simulink model "FeedbackData"  (Simulink 7.6)
settings: Solver=FixedStepDiscrete  StartTime=0.0  StopTime=runTime  FixedStep=dt  RelTol=1e-3
values from neighbouring files (symbols this model uses):
  dataSize = hmDataSize + rigidBodies*rigidBodyDataSize + markers*markerDataSize    (= 111)    [initCode.m]
  dt = 1/52    (= 0.0192307692308)    [initCode.m]    (also in logdata.m)
  hypx = modeldata.muscle(10).Fx.hyp.cov    [initCode.m]
  hypy = modeldata.muscle(10).Fy.hyp.cov    [initCode.m]
  hypz = modeldata.muscle(10).Fz.hyp.cov    [initCode.m]
  Ki = 0    [initCode.m]
  Kp = 0    [initCode.m]
  KXX_x = (KXX+sigma2*eye(size(KXX,1)))    [initCode.m]
  KXX_y = (KXX+sigma2*eye(size(KXX,1)))    [initCode.m]
  KXX_z = (KXX+sigma2*eye(size(KXX,1)))    [initCode.m]
  M = data(idx).M    [initCode.m]
  maxF = [max(trainingOutputs_x),max(trainingOutputs_y),max(trainingOutputs_z)]    [initCode.m]
  minF = [min(trainingOutputs_x),min(trainingOutputs_y),min(trainingOutputs_z)]    [initCode.m]
  pwmat = [0 0 0 0 0 0 0 0 0;250 23 10 20 49 62 107 22 25]    [initCode.m]
  rcparams = zeros(9,4)    [initCode.m]
  runTime = 5    [initCode.m]
  stimStartTime = 0.1    [initCode.m]
  trainingInputs = modeldata.muscle(10).Fx.trainingInputs    [initCode.m]
  trainingOutputs_x = modeldata.muscle(10).Fx.trainingOutputs    [initCode.m]
  trainingOutputs_y = modeldata.muscle(10).Fy.trainingOutputs    [initCode.m]
  trainingOutputs_z = modeldata.muscle(10).Fz.trainingOutputs    [initCode.m]
  trajectory = [data(idx).traj(:,1:3) data(idx).t(:,1:3) data(idx).forceRange]    [initCode.m]
undefined symbols (not defined in the file or in its folder): DiscIntNeverNeededParam, Implant, IST
libraries: xpclib x8, devices x5, FreqBlockset x2, simulink x1
settings Model: Creator=Engineer  LastModifiedBy=KirschLab  BufferReuse=off
settings DataIOCC: LimitDataPoints=off  SaveFormat=StructureWithTime  SignalLogging=off
settings OptimizationCC: BlockReduction=off  OptimizeBlockIOStorage=off  BufferReuse=off  ExpressionFolding=off  LocalBlockOutputs=off  InitFltsAndDblsToZero=on  SimCompilerOptimization=On
settings DebuggingCC: StrictBusMsg=Warning
settings HardwareCC: ProdIntDivRoundTo=Zero  ProdEndianess=LittleEndian  ProdHWDeviceType=Generic->32-bit x86 compatible  TargetHWDeviceType=32-bit Generic
settings RTWCC: SystemTargetFile=xpctarget.tlc  TemplateMakefile=xpc_default_tmf  Description=xPC Target  ProcessScript=xpctarget_make_rtw_hook  RTWCompilerOptimization=On
settings xpcTargetCC: TargetFcnLib=ansi_tfl_table_tmw.mat  TargetFunctionLibrary=XPC_BLAS  ERTCodeCoverageTool=None  ParMdlRefBuildCompliant=on  CombineSignalStateStructs=off  PortableWordSizes=off  xPCLoadParamSetFile=off  xPCConcurrentTasks=off  xPCEnableSFAnimation=off

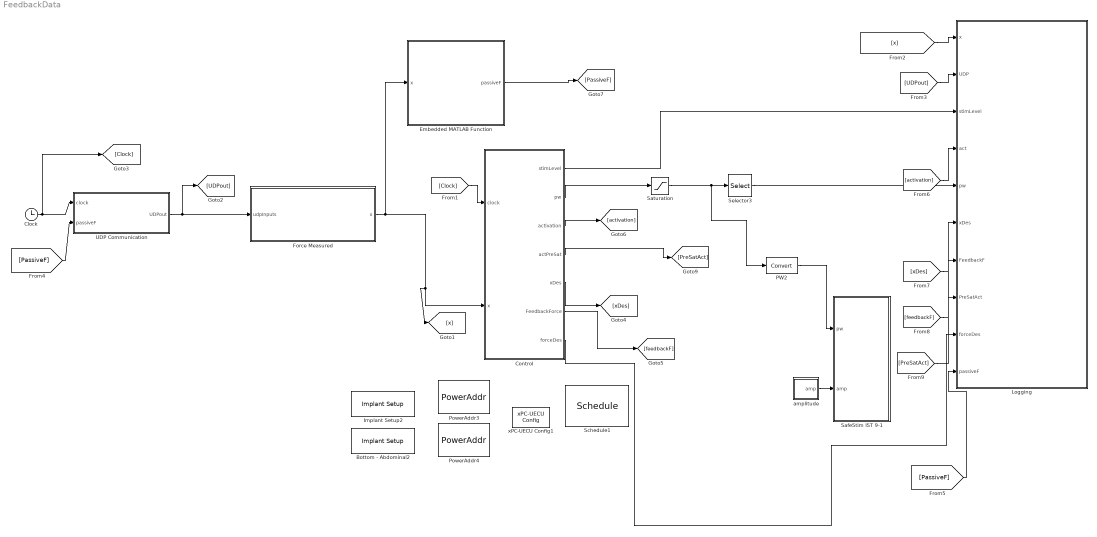
== system FeedbackData ==
  Bottom - Abdominal2 : devices/Implant Setup  implant=IST-12  addr=Implant(2).Addr  port=Implant(2).Port  id=0  hs=off  dup=off
  Clock : Clock
      settings: Decimation=10
  Control : Subsystem  TreatAsAtomicUnit=on
  Embedded MATLAB Function : Stateflow chart  TreatAsAtomicUnit=on
  Force Measured : Subsystem
  Implant Setup2 : devices/Implant Setup  implant=IST-12  addr=Implant(1).Addr  port=Implant(1).Port  id=0  hs=off  dup=off
  Logging : Subsystem
  PW2 : DataTypeConversion
  PowerAddr3 : FreqBlockset/Schedule_Setup/PowerAddr  SystemSampleTime=-1  rf_power=Implant(1).Power  addr=Implant(1).Addr  sched_T=uecuFreq  port=Implant(1).Port
  PowerAddr4 : FreqBlockset/Schedule_Setup/PowerAddr  SystemSampleTime=-1  rf_power=Implant(2).Power  addr=Implant(2).Addr  sched_T=uecuFreq  port=Implant(2).Port
  SafeStim IST 9-1 : Subsystem  mask{addr=Implant(2).Addr, port=Implant(2).Port, chvector=[0 1 2 3 4 5 6 7 8 9 10 11], alimits=[4 4 2 3 2 3 2 2 3 5 5 8], dvector=[10 11 12 13 14 15 16 17 18 19 20 21], schedulename=schedule1, spriority=100, Tsamp=-1}
      mask prompts: addr "Address"; chvector "Channel Vector"; alimits "Amplitude Level Limits"; dvector "Delay vector (ms)"; schedulename "Schedule name"; spriority "Scheduler priority"; Tsamp "Sample time (s) (Update rate.  Pulse period is set by Schedule block.)"
      mask CallbackString: |||||set_param([gcb '/Stim'],'sched',get_param(gcb,'schedulename'))||
      mask Display:
      | fprintf('Safe Stimulation\nSet Amp Limits')
      | port_label('input',1,'pw(us)')
      | port_label('input',2,'amp(level)')
  Saturation : Saturate  UpperLimit=250  LowerLimit=0
  Schedule1 : devices/Schedule  sched=schedule1  stype=Synchronous  period=80  t=1/13
  Selector3 : Selector  InputPortWidth=12  IndexOptions=Index vector (dialog)  Indices=[1 2 3 4 7 9 10 11 12]  OutputSizes=1
  UDP Communication : Subsystem
  amplitude : Subsystem
  xPC-UECU Config1 : devices/xPC Functions/xPC-UECU Config  port=COM1  baud=115200  flowctrl=on  addr=128
  wires:
  [UDPout] -> Logging/2(UDP)
  Control/1(stimLevel) -> Logging/3(stimLevel)
  Control/2(pw) -> Saturation/1
  Saturation/1 -> PW2/1, Selector3/1
  [Clock] -> Control/1(clock)
  Control/3(activation) -> [activation]
  PW2/1 -> SafeStim IST 9-1/1(pw)
  amplitude/1(amp) -> SafeStim IST 9-1/2(amp)
  [x] -> Logging/1(x)
  [activation] -> Logging/4(act)
  Selector3/1 -> Logging/5(pw)
  UDP Communication/1(UDPout) -> [UDPout], Force Measured/1(udpInputs)
  Clock/1 -> UDP Communication/1(clock), [Clock]
  [feedbackF] -> Logging/7(FeedbackF)
  [xDes] -> Logging/6(xDes)
  Control/4(actPreSat) -> [PreSatAct]
  [PreSatAct] -> Logging/8(PreSatAct)
  Control/5(xDes) -> [xDes]
  Force Measured/1(x) -> Control/2(x), [x], Embedded MATLAB Function/1(x)
  Control/6(FeedbackForce) -> [feedbackF]
  Control/7(forceDes) -> Logging/9(forceDes)
  Embedded MATLAB Function/1(passiveF) -> [PassiveF]
  [PassiveF] -> UDP Communication/2(passiveF)
  [PassiveF] -> Logging/10(passiveF)

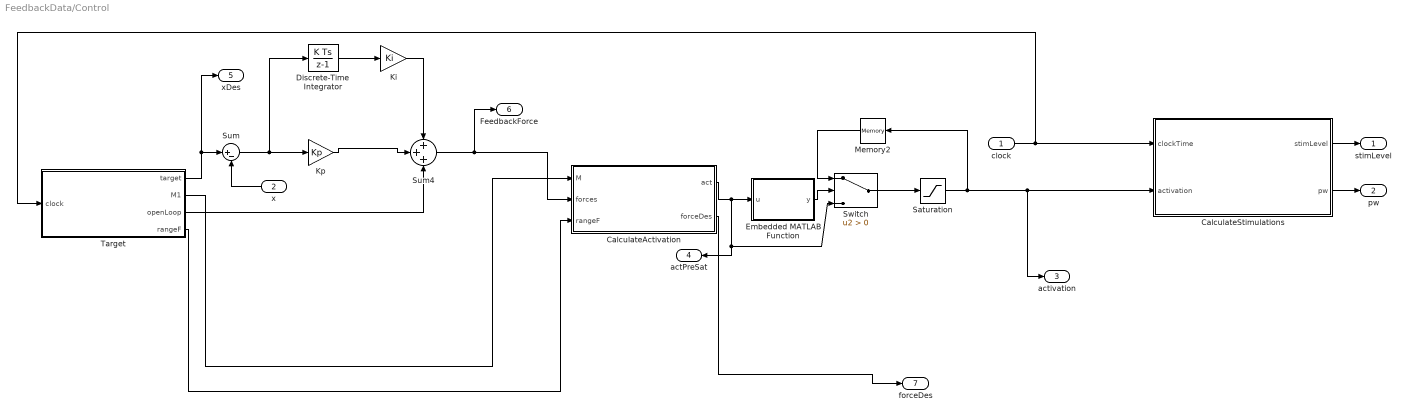
== system FeedbackData/Control ==
  clock : Inport
  x : Inport  Port=2
  CalculateActivation : Stateflow chart  TreatAsAtomicUnit=on
  CalculateStimulations : Stateflow chart  TreatAsAtomicUnit=on
  Discrete-Time Integrator : DiscreteIntegrator  InitialCondition=[0;0;0]  SampleTime=dt  LimitOutput=on  UpperSaturationLimit=[50;50;50]  LowerSaturationLimit=[-50;-50;-50]  ICPrevOutput=DiscIntNeverNeededParam  ICPrevScaledInput=DiscIntNeverNeededParam
  Embedded MATLAB Function : Stateflow chart  TreatAsAtomicUnit=on
  Ki : Gain  Gain=Ki
  Kp : Gain  Gain=Kp
  Memory2 : Memory  X0=[0;0;0;0;0;0;0;0;0]
  Saturation : Saturate  UpperLimit=1  LowerLimit=0
  Sum : Sum  Inputs=|+-
  Sum4 : Sum  Inputs=+++
  Switch : Switch  Criteria=u2 > Threshold
  Target : Stateflow chart  TreatAsAtomicUnit=on
  stimLevel : Outport
  pw : Outport  Port=2
  activation : Outport  Port=3
  actPreSat : Outport  Port=4
  xDes : Outport  Port=5
  FeedbackForce : Outport  Port=6
  forceDes : Outport  Port=7
  wires:
  CalculateStimulations/2(pw) -> pw/1
  CalculateStimulations/1(stimLevel) -> stimLevel/1
  clock/1 -> CalculateStimulations/1(clockTime), Target/1(clock)
  CalculateActivation/1(act) -> Switch/3, actPreSat/1, Embedded MATLAB Function/1(u)
  Saturation/1 -> activation/1, CalculateStimulations/2(activation), Memory2/1
  Memory2/1 -> Switch/1
  Embedded MATLAB Function/1(y) -> Switch/2
  Switch/1 -> Saturation/1
  Target/1(target) -> Sum/1, xDes/1
  x/1 -> Sum/2
  Sum/1 -> Kp/1, Discrete-Time Integrator/1
  Discrete-Time Integrator/1 -> Ki/1
  Ki/1 -> Sum4/1
  Kp/1 -> Sum4/2
  Sum4/1 -> CalculateActivation/2(forces), FeedbackForce/1
  Target/2(M1) -> CalculateActivation/1(M)
  Target/3(openLoop) -> Sum4/3
  Target/4(rangeF) -> CalculateActivation/3(rangeF)
  CalculateActivation/2(forceDes) -> forceDes/1

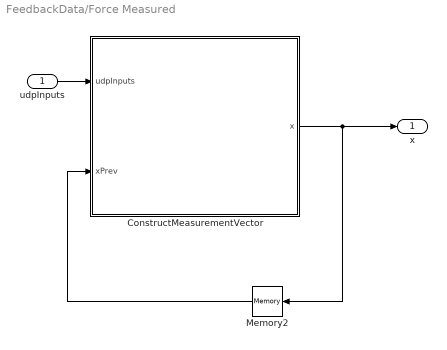
== system FeedbackData/Force Measured ==
  udpInputs : Inport
  ConstructMeasurementVector : Stateflow chart  TreatAsAtomicUnit=on
  Memory2 : Memory  X0=[0;0;0]
  x : Outport
  wires:
  udpInputs/1 -> ConstructMeasurementVector/1(udpInputs)
  ConstructMeasurementVector/1(x) -> x/1, Memory2/1
  Memory2/1 -> ConstructMeasurementVector/2(xPrev)

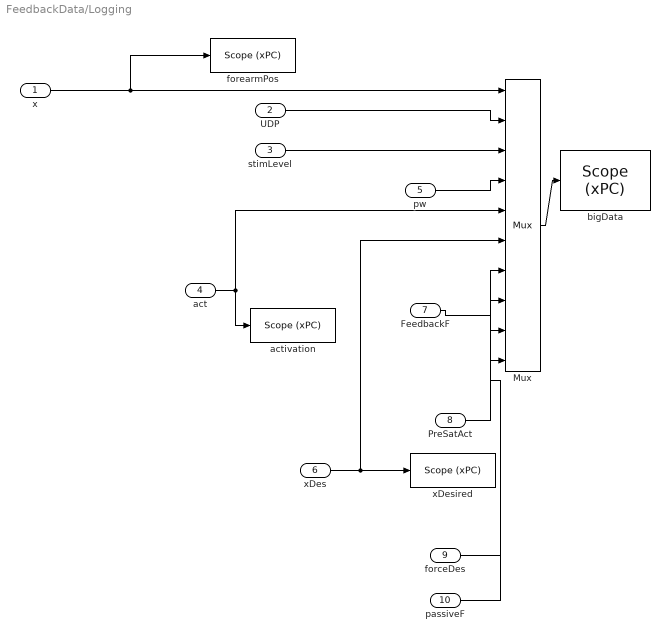
== system FeedbackData/Logging ==
  x : Inport
  UDP : Inport  Port=2
  stimLevel : Inport  Port=3
  act : Inport  Port=4
  pw : Inport  Port=5
  xDes : Inport  Port=6
  FeedbackF : Inport  Port=7
  PreSatAct : Inport  Port=8
  forceDes : Inport  Port=9
  passiveF : Inport  Port=10
  Mux : Mux  Inputs=10
  activation : xpclib/Misc./Scope (xPC)   SystemSampleTime=-1  scopeno=5  scopetype=Target  autostart=on  viewmode=Numerical  formatstr='%15.6f'  grid=on  ylimits=[-1,1]  nosamples=3  noprepostsamples=-50  interleave=1  triggermode=FreeRun  triggersignal=2  triggerlevel=0.5  triggerslope=Either  triggerscope=1  triggersample=0  filename=data.dat  mode=Lazy  writesize=512  autorestart=off  dynamicfilemode=off  maxwritefilesize=512*1024^2
  bigData : xpclib/Misc./Scope (xPC)   SystemSampleTime=-1  scopeno=1  scopetype=File  autostart=on  viewmode=Numerical  formatstr='%15.6f'  grid=on  ylimits=[-1,1]  nosamples=10000  noprepostsamples=-50  interleave=dec  triggermode=FreeRun  triggersignal=2  triggerlevel=0.5  triggerslope=Either  triggerscope=1  triggersample=0  filename=data3.dat  mode=Lazy  writesize=512  autorestart=off  dynamicfilemode=off  maxwritefilesize=512*1024^2
  forearmPos : xpclib/Misc./Scope (xPC)   SystemSampleTime=-1  scopeno=3  scopetype=Target  autostart=on  viewmode=Numerical  formatstr='%15.6f'  grid=on  ylimits=[-1,1]  nosamples=3  noprepostsamples=-50  interleave=1  triggermode=FreeRun  triggersignal=2  triggerlevel=0.5  triggerslope=Either  triggerscope=1  triggersample=0  filename=data.dat  mode=Lazy  writesize=512  autorestart=off  dynamicfilemode=off  maxwritefilesize=512*1024^2
  xDesired : xpclib/Misc./Scope (xPC)   SystemSampleTime=-1  scopeno=4  scopetype=Target  autostart=on  viewmode=Numerical  formatstr='%15.6f'  grid=on  ylimits=[-1,1]  nosamples=3  noprepostsamples=-50  interleave=1  triggermode=FreeRun  triggersignal=2  triggerlevel=0.5  triggerslope=Either  triggerscope=1  triggersample=0  filename=data.dat  mode=Lazy  writesize=512  autorestart=off  dynamicfilemode=off  maxwritefilesize=512*1024^2
  wires:
  act/1 -> activation/1, Mux/5
  pw/1 -> Mux/4
  Mux/1 -> bigData/1
  x/1 -> Mux/1, forearmPos/1
  UDP/1 -> Mux/2
  stimLevel/1 -> Mux/3
  xDes/1 -> xDesired/1, Mux/6
  FeedbackF/1 -> Mux/7
  PreSatAct/1 -> Mux/8
  forceDes/1 -> Mux/9
  passiveF/1 -> Mux/10

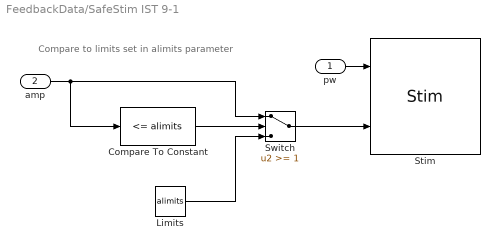
== system FeedbackData/SafeStim IST 9-1 ==
  note: Compare to limits set in alimits parameter
  pw : Inport
  amp : Inport  Port=2
  Compare To Constant : simulink/Logic and Bit Operations/Compare To Constant  SystemSampleTime=-1  relop=<=  const=alimits  LogicOutDataTypeMode=uint8  ZeroCross=off
  Limits : Constant  Value=alimits  OutDataTypeStr=uint8  SampleTime=Tsamp
  Stim : devices/Stim  addr=addr  port=port  chan=chvector  dselect=Parameter  delays=dvector  autosched=Manual  sched=schedule1  pri=spriority  period=Tsamp
  Switch : Switch  Threshold=1  SampleTime=Tsamp
  wires:
  pw/1 -> Stim/1
  amp/1 -> Compare To Constant/1, Switch/1
  Compare To Constant/1 -> Switch/2
  Limits/1 -> Switch/3
  Switch/1 -> Stim/2

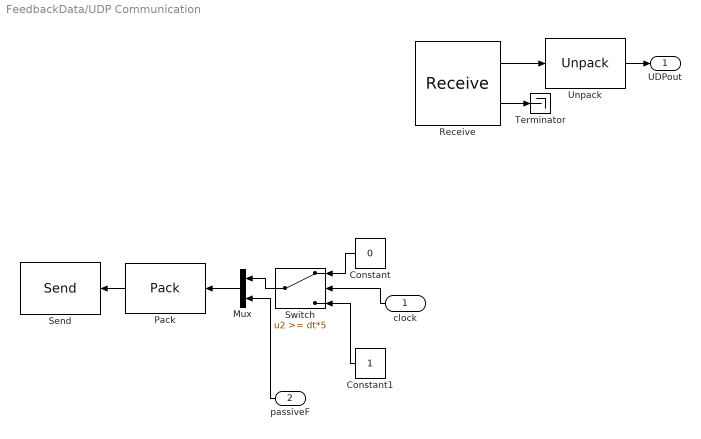
== system FeedbackData/UDP Communication ==
  clock : Inport
  passiveF : Inport  Port=2
  Constant : Constant  Value=0
  Constant1 : Constant
  Mux : Mux  Inputs=2
  Pack : xpclib/UDP/Pack  datatypes={'double'}  byteAlign=1
  Receive : xpclib/UDP/Receive  ipAddress=192.168.0.8  ipPort=25000  width=8*dataSize  vblLen=off  sampletime=dt
  Send : xpclib/UDP/Send  ipAddress=192.168.0.8  ipPort=20000  localPort=-1  vblLen=off  sampletime=dt
  Switch : Switch  Threshold=dt*5
  Terminator : Terminator
  Unpack : xpclib/UDP/Unpack  dimensions={[dataSize]}  datatypes={'double'}  byteAlign=1
  UDPout : Outport
  wires:
  Receive/2 -> Terminator/1
  Receive/1 -> Unpack/1
  Pack/1 -> Send/1
  clock/1 -> Switch/2
  Constant/1 -> Switch/1
  Constant1/1 -> Switch/3
  Unpack/1 -> UDPout/1
  Mux/1 -> Pack/1
  Switch/1 -> Mux/1
  passiveF/1 -> Mux/2

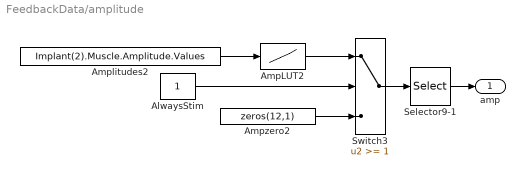
== system FeedbackData/amplitude ==
  AlwaysStim : Constant
  AmpLUT2 : Lookup  InputValues=Implant(2).Muscle.Amplitude.AmpIndices(:,1)  Table=Implant(2).Muscle.Amplitude.AmpIndices(:,2)  LookUpMeth=Interpolation-Use End Values  OutDataTypeStr=uint8  SaturateOnIntegerOverflow=on
  Amplitudes2 : Constant  Value=Implant(2).Muscle.Amplitude.Values  OutDataTypeStr=double
  Ampzero2 : Constant  Value=zeros(12,1)  OutDataTypeStr=uint8
  Selector9-1 : Selector  InputPortWidth=12  IndexOptions=Index vector (dialog)  Indices=[1 2 3 4 5 6 7 8 9 10 11 12]  OutputSizes=1
  Switch3 : Switch  Threshold=1
  amp : Outport
  wires:
  Amplitudes2/1 -> AmpLUT2/1
  Ampzero2/1 -> Switch3/3
  Switch3/1 -> Selector9-1/1
  AmpLUT2/1 -> Switch3/1
  AlwaysStim/1 -> Switch3/2
  Selector9-1/1 -> amp/1

== matlab function Control/Embedded MATLAB Function ==
  data: u input double; y output double
function y = fcn(u)
%#eml

y = sum(isnan(u));

== matlab function Control/Target ==
  data: trajectory parameter double; M parameter double; target output double; clock input double; runTime parameter double; M1 output double; openLoop output double; rangeF output double
function [target,M1,openLoop,rangeF]   = calcTarget(trajectory,M,clock,runTime)
%#eml

dt=1/52;
steps=runTime/dt;
idx=floor(clock/runTime*steps)+1;
if idx>length(trajectory)
    idx=length(trajectory);
end


target=trajectory(idx,1:3)';
openLoop=trajectory(idx,4:6)';
M1=M(:,:,idx);
rangeF=trajectory(idx,7:12)';

== matlab function Force Measured/ConstructMeasurementVector ==
  data: udpInputs input double; x output double; xPrev input double
function x    = cmv(udpInputs,xPrev)
%#eml


forearmFlagIndex = 39;

forearmFlag = udpInputs(forearmFlagIndex); 
if forearmFlag % if the forearm rigid body is visiable record the sensor readings
	x = udpInputs(36:38); 
else 
    x=xPrev;
end

== matlab function Control/CalculateActivation ==
  data: M input double; act output double; forces input double; actDesired parameter double; rangeF input double; forceDes output double
function [act,forceDes]  = computeActivations(M,forces,actDesired,rangeF)
%#eml

% % solve Malpha=forces for alpha


% Use desired activation if previous activations were too high or low
% This should help stop the solution from running away

x=actDesired;
normal = [0 0 1; 0 0 -1; -1 0 0; 1 0 0; 0 1 0; 0 -1 0];

forceDes=forces;
Fdes=forceDes;
unitvector=Fdes';
% Make norm of forces small if needed
% Method by Zinnia Hall
xyz_max=rangeF([2 4 6]);
xyz_min=rangeF([1 3 5]);
if Fdes(1)> xyz_max(1) || Fdes(2)> xyz_max(2) || Fdes(3)> xyz_max(3) || Fdes(1)< xyz_min(1) || Fdes(2)< xyz_min(2) || Fdes(3)< xyz_min(3)
    xyz_plane1 = [xyz_min(1) xyz_min(2) xyz_max(3)];
    xyz_plane2 = [xyz_min(1) xyz_min(2) xyz_min(3)];
    xyz_plane3 = [xyz_min(1) xyz_max(2) xyz_max(3)];
    xyz_plane4 = [xyz_max(1) xyz_min(2) xyz_min(3)];
    xyz_plane5 = [xyz_max(1) xyz_max(2) xyz_max(3)];
    xyz_plane6 = [xyz_max(1) xyz_min(2) xyz_max(3)];
    d1 = (dot((xyz_plane1 - zeros(1,3)),normal(1,:)))/(dot(unitvector,normal(1,:)));
    d2 = (dot((xyz_plane2 - zeros(1,3)),normal(2,:)))/(dot(unitvector,normal(2,:)));
    d3 = (dot((xyz_plane3 - zeros(1,3)),normal(3,:)))/(dot(unitvector,normal(3,:)));
    d4 = (dot((xyz_plane4 - zeros(1,3)),normal(4,:)))/(dot(unitvector,normal(4,:)));
    d5 = (dot((xyz_plane5 - zeros(1,3)),normal(5,:)))/(dot(unitvector,normal(5,:)));
    d6 = (dot((xyz_plane6 - zeros(1,3)),normal(6,:)))/(dot(unitvector,normal(6,:)));
    % ratio of perpendicular distance between point on plane vector and infeasible vector
    distance = [d1 d2 d3 d4 d5 d6];
    distance = distance(distance>=0); %creates vector with positive values
    distance = min(distance);
    point = (distance*unitvector)+zeros(1,3);
    Fdes_new = point; % Point of intersection with plane
    forceDes=Fdes_new';
end

forces=forceDes;
Bk=eye(9);
func=@penaltyFunc;
[f,g]=func(x,M,forces);

it=0;
while norm(g)>1e-3 && it<120
    p=-Bk*g;
    alpha2=armijo(func,x,f,g,p,M,forces);
    xold=x;
    x=x+alpha2*p;
    sk=x-xold;
    gold=g;
    [f,g]=func(x,M,forces);
    yk=g-gold;
    rho=1/(yk'*sk);
    Bk=(eye(9)-rho*sk*yk')*Bk*(eye(9)-rho*yk*sk')+rho*sk*sk';
    it=it+1;
end

if max(x)>1
    x=x/max(x);
end


act=x;
end

function alpha1 = armijo(func,xk,fk,gradk,pk,M,forces)
% Originally from Dr. Schearer. Modified by Derek Wolf
alpha1   = 1;
c       = 0;
rho     = 0.5;

n=0;
while fk + c*alpha1*gradk'*pk < func(xk+alpha1*pk,M,forces) % sufficient descent condition is not met
    alpha1 = rho*alpha1;
    n=n+1;
end
end

function [f,g]=penaltyFunc(x,M,forces)
c3 = 1000;
c2 = 10000;
c1 = 100;

K=0;
for i=1:length(x)
    if x(i)<0
        K=K+x(i)^2;
    end
    if x(i)>1
        K = K + (x(i)-1)^2;
    end
end

dirConst = [forces(2)*M(3,:)-forces(3)*M(2,:);forces(3)*M(1,:)-forces(1)*M(3,:);forces(1)*M(2,:)-forces(2)*M(1,:)];
f=norm(x)^2+c1*norm(M*x-forces)^2+c2*K + c3*norm(dirConst*x)^2;

if nargout>1
    % Define gradient
    K=zeros(9,1);
    for i=1:length(x)
        if x(i)<0
            K(i)=2*x(i);
        end
        if x(i) > 1
            K(i) = 2*(x(i)-1);
        end
    end
    
    g = 2*x + 2*c1*M'*(M*x-forces) + c2*K + 2*c3*dirConst'*dirConst*x;
end


end

% function [f,g]=penaltyFunc(x,M,forces)
%
% c2=5000;
% c=1;
%
%
% K=0;
% for i=1:length(x)
%     if x(i)<0
%         K=K+x(i)^2;
%     end
% end
%
% f=c*norm(x)^2+norm(M*x-forces)^2+c2*K;
%
% if nargout>1
%     % Define gradient
%     K=zeros(9,1);
%     for i=1:length(x)
%         if x(i)<0
%             K(i)=2*x(i);
%         end
%     end
%
%     g=c*2*x+2*M'*(M*x-forces)+c2*K;
% end
%
%
% end
%
%
%

== matlab function Control/CalculateStimulations ==
  data: pwmat parameter double; runTime parameter double; rcparams parameter double; stimStartTime parameter double; clockTime input double; activation input double; stimLevel output double; pw output double
function [stimLevel,pw] = calcStims(pwmat,runTime,rcparams,stimStartTime,clockTime,activation)
%#eml

activation=activation';
stimulations=zeros(1,9);
for k = 1:9 % loop though muscles
    biasTerm = rcparams(k,1)/(1+exp(rcparams(k,2)*(rcparams(k,3)-0)));
    forceAT100 = rcparams(k,1)/(1+exp(rcparams(k,2)*(rcparams(k,3)-1))) - biasTerm;
    stimulations(:,k) = rcparams(k,3) - log(rcparams(k,1)./(forceAT100*activation(:,k)+biasTerm)-1)./rcparams(k,2);
end

stim = stimulations;

if clockTime>stimStartTime && clockTime<=runTime-0.2  % Send zero at end and 0 if error is greater than 25 cm
    stimulations = zeros(9,1);
    for i = 1:9
       stimulations(i) = pwmat(1,i) + stim(i)*(pwmat(2,i)-pwmat(1,i));
    end
else
    stim=zeros(1,9);
    stimulations=zeros(9,1);
end


stimLevel = stim;
pw = floor([stimulations(1) stimulations(2) stimulations(3) stimulations(4) 0 0 stimulations(5) 0 stimulations(6) stimulations(7) stimulations(8) stimulations(9)]');

== matlab function Embedded MATLAB Function ==
  data: hypx parameter double; hypy parameter double; hypz parameter double; passiveF output double; KXX_x parameter double; KXX_y parameter double; KXX_z parameter double; trainingInputs parameter double; trainingOutputs_x parameter double; trainingOutputs_y parameter double; trainingOutputs_z parameter double; maxF parameter double; minF parameter double; x input double
function passiveF = PassiveForceCalc(hypx,hypy,hypz,KXX_x,KXX_y,KXX_z,trainingInputs,trainingOutputs_x,trainingOutputs_y,trainingOutputs_z,maxF,minF,x)
%#eml

q=x';

% Required force in x direction
K_xsX=covSEard_realTime(hypx,trainingInputs,q);
Fx=K_xsX'/KXX_x*trainingOutputs_x;

K_xsX=covSEard_realTime(hypy,trainingInputs,q);
Fy=K_xsX'/KXX_y*trainingOutputs_y;

K_xsX=covSEard_realTime(hypz,trainingInputs,q);
Fz=K_xsX'/KXX_z*trainingOutputs_z;

passiveF = [Fx,Fy,Fz];

for dof=1:3
    if passiveF(dof)>maxF(dof)
        passiveF(dof)=maxF(dof);
    elseif passiveF(dof)<minF(dof)
        passiveF(dof)=minF(dof);
    end
end
